simulink model "robot_etu"  (R2021b)
settings: Solver=VariableStepAuto  StartTime=0.0  StopTime=10.0  RelTol=1e-3
values from neighbouring files (symbols this model uses):
  K = -place(A,B,poles)    [matrices.m]    (also in simu_robot_etu.m = [0.6700 19.9055 1.0747 1.9614])
  ue = 0    [simu_robot_etu.m]
  x0 = [0 pi/10 0 0]    [simu_robot_etu.m]
  xe = [0 0 0 0]'    [simu_robot_etu.m]
settings Model: Creator=ialouane  LastModifiedBy=ialouane

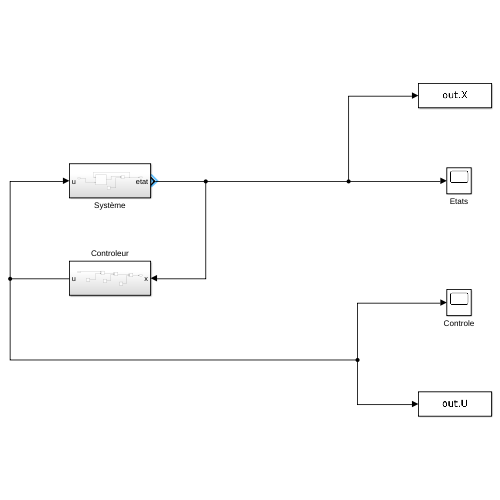
[thumbnail: Simulink's stored preview of the top-level diagram]
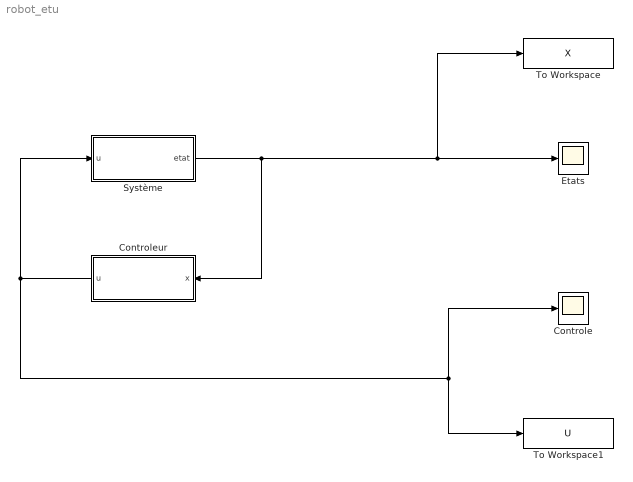
== system robot_etu ==
  Controle : Scope
  Controleur : Subsystem
  Etats : Scope
  Système : Subsystem
  To Workspace : ToWorkspace  VariableName=X  SaveFormat=Timeseries  SampleTime=-1
  To Workspace1 : ToWorkspace  VariableName=U  SaveFormat=Timeseries  SampleTime=-1
  wires:
  Système/1(etat) -> To Workspace/1, Etats/1, Controleur/1(x)
  Controleur/1(u) -> Système/1(u), To Workspace1/1, Controle/1

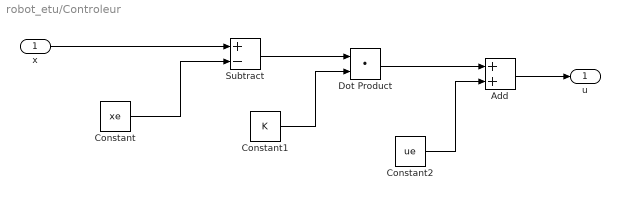
== system robot_etu/Controleur ==
  x : Inport
  Add : Sum
  Constant : Constant  Value=xe
  Constant1 : Constant  Value=K  VectorParams1D=off
  Constant2 : Constant  Value=ue
  Dot Product : DotProduct  InputSameDT=on  OutDataTypeStr=Inherit: Inherit via internal rule
  Subtract : Sum  Inputs=+-
  u : Outport
  wires:
  Add/1 -> u/1
  Constant2/1 -> Add/2
  Dot Product/1 -> Add/1
  Constant1/1 -> Dot Product/2
  Subtract/1 -> Dot Product/1
  Constant/1 -> Subtract/2
  x/1 -> Subtract/1

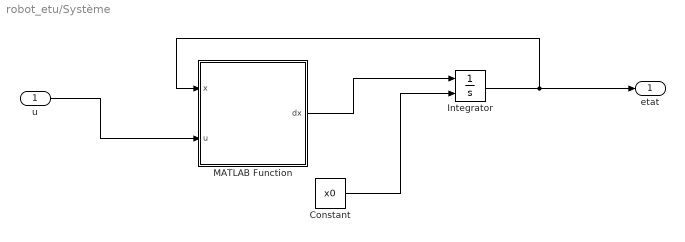
== system robot_etu/Système ==
  u : Inport
  Constant : Constant  Value=x0
  Integrator : Integrator  InitialConditionSource=external
  MATLAB Function : MATLAB Function  TreatAsAtomicUnit=on
  etat : Outport
  wires:
  u/1 -> MATLAB Function/2(u)
  MATLAB Function/1(dx) -> Integrator/1
  Constant/1 -> Integrator/2
  Integrator/1 -> MATLAB Function/1(x), etat/1

== matlab function robot_etu/Système/MATLAB Function ==
  data: x input; u input; dx output
function dx = fcn( x, u)
dx = fonction(x,u);
end
